simulink model "PVarray_Grid_IncCondReg_det"  (Simulink 10.1)
settings: Solver=FixedStepDiscrete  StartTime=0.0  StopTime=3  RelTol=1e-3
PreLoadFcn:
  | Ts_Power=1e-6
  | Ts_Control=100e-6
undefined symbols (not defined in the file or in its folder): D1, Delta, DiscIntNeverNeededParam, level, sigbuilder_block
libraries: powerlib x29, powerlib_extras x7, simulink x4
(part 2 of 2)

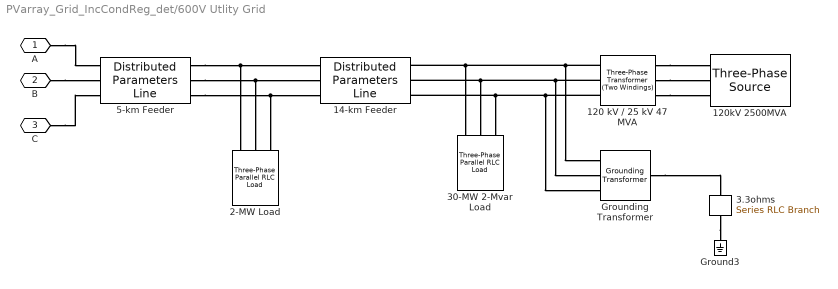
== system PVarray_Grid_IncCondReg_det/600V Utlity Grid ==
  120 kV / 25 kV 47 MVA : powerlib/Elements/Three-Phase Transformer (Two Windings)  Winding1Connection=Yg  Winding2Connection=Delta (D1)  CoreType=Three single-phase transformers  SetSaturation=off  Hysteresis=off  DataFile='basic_model'  SetInitialFlux=off  Measurements=None  UNITS=pu  NominalPower=[47e6 60 ]  Winding1="[ 120e3  0.08/30   0.08 ]"  Winding2="[ 25e3  0.08/30  0.08]"  Rm=500  Lm=500  L0=0.5  Saturation="[ 0,0  ;  0.005,1.2  ;  1.0,1.4 ]"  InitialFluxes=[ 0.8 , -0.8 , 0.7 ]  BreakLoop=off  DiscreteSolver=Trapezoidal iterative  DataType=off  TransfoNumber=0
  120kV 2500MVA : powerlib/Electrical Sources/Three-Phase Source  InternalConnection=Yg  VoltagePhases=off  Voltage=120e3  PhaseAngle=0  Voltage_phases=[25e3 25e3 25e3]/sqrt(3)  PhaseAngles_phases=[0 -120 +120]  Frequency=60  NonIdealSource=on  SpecifyImpedance=on  Resistance=0.8929  Inductance=16.58e-3  ShortCircuitLevel=2500e6  BaseVoltage=120e3  XRratio=7  BusType=swing  Pref=0  Qref=0  Prefabc=[10e3, 10e3, 10e3]  Qrefabc=[0, 0, 0]  Qmin=-inf  Qmax=inf
  14-km Feeder : powerlib/Elements/Distributed Parameters Line  Phases=3  Frequency=60  Resistance=[0.1153 0.413]  Inductance=[1.05e-3 3.32e-3]  Capacitance=[11.33e-009 5.01e-009]  Length=14  x1=[-5.8e-05 -8.79995943472587e-10 0 0;-5.7e-05 -8.80194503979229e-10 0 0;-5.6e-05 -8.80392939390602e-10 0 0;-5.5e-05 -8.80591249678504e-10 0 0;-5.4e-05 -8.80789434814751e-10 0 0;-5.3e-05 -8.80987494771175e-10 0 0;-5.2e-05 -8.8118542951963e-10 0 0;-5.1e-05 -8.81383239031983e-10 0 0;-5e-05 -8.81580923280121e-10 0 0;-4.9e-05 -8.8177848223595e-10 -3790.5008820983 -24060.9143986483;-4.8e-05 -8.81975915871391e-10 -3781.42986192619 -24062.3416739851;-4.7e-05 -8.82173224158384e-10 -3772.35830432856 -24063.7655295266;-4.6e-05 -8.82370407068889e-10 -3763.28621059469 -24065.1859650703;-4.5e-05 -8.8256746457488e-10 -3754.21358201392 -24066.6029804144;-4.4e-05 -8.82764396648352e-10 -3745.14041987568 -24068.0165753574;-4.3e-05 -8.82961203261316e-10 -3736.06672546945 -24069.4267496986;-4.2e-05 -8.83157884385802e-10 -3726.99250008483 -24070.8335032374;-4.1e-05 -8.83354439993856e-10 -3717.91774501146 -24072.236835774;-4e-05 -8.83550870057544e-10 -3708.84246153905 -24073.6367471089;-3.9e-05 -8.83747174548949e-10 -3699.76665095742 -24075.0332370431;-3.8e-05 -8.83943353440171e-10 -3690.69031455644 -24076.4263053782;-3.7e-05 -8.84139406703329e-10 -3681.61345362605 -24077.8159519161;-3.6e-05 -8.8433533431056e-10 -3672.53606945629 -24079.2021764594;-3.5e-05 -8.84531136234017e-10 -3663.45816333725 -24080.5849788111;-3.4e-05 -8.84726812445874e-10 -3654.3797365591 -24081.9643587746;-3.3e-05 -8.84922362918319e-10 -3645.30079041209 -24083.3403161539;-3.2e-05 -8.85117787623562e-10 -3636.22132618654 -24084.7128507535;-3.1e-05 -8.85313086533827e-10 -3627.14134517285 -24086.0819623782;-3e-05 -8.85508259621359e-10 -3618.06084866149 -24087.4476508336;-2.9e-05 -8.85703306858418e-10 -3608.97983794298 -24088.8099159254;-2.8e-05 -8.85898228217286e-10 -3599.89831430796 -24090.1687574601;-2.7e-05 -8.86093023670258e-10 -3590.8162790471 -24091.5241752446;-2.6e-05 -8.86287693189649e-10 -3581.73373345117 -24092.8761690862;-2.5e-05 -8.86482236747794e-10 -3572.65067881099 -24094.2247387928;-2.4e-05 -8.86676654317043e-10 -3563.56711641748 -24095.5698841727;-2.3e-05 -8.86870945869765e-10 -3554.4830475616 -24096.9116050348;-2.2e-05 -8.87065111378347e-10 -3545.39847353442 -24098.2499011883;-2.1e-05 -8.87259150815193e-10 -3536.31339562704 -24099.5847724431;-2e-05 -8.87453064152727e-10 -3527.22781513066 -24100.9162186094;-1.9e-05 -8.87646851363389e-10 -3518.14173333655 -24102.2442394981;-1.8e-05 -8.87840512419637e-10 -3509.05515153604 -24103.5688349203;-1.7e-05 -8.88034047293948e-10 -3499.96807102053 -24104.8900046878;-1.6e-05 -8.88227455958816e-10 -3490.8804930815 -24106.2077486129;-1.5e-05 -8.88420738386753e-10 -3481.79241901051 -24107.5220665083;-1.4e-05 -8.88613894550291e-10 -3472.70385009916 -24108.8329581871;-1.3e-05 -8.88806924421976e-10 -3463.61478763914 -24110.1404234631;-1.2e-05 -8.88999827974376e-10 -3454.52523292222 -24111.4444621504;-1.1e-05 -8.89192605180074e-10 -3445.43518724023 -24112.7450740638;-1e-05 -8.89385256011672e-10 -3436.34465188505 -24114.0422590183;-9e-06 -8.8957778044179e-10 -3427.25362814866 -24115.3360168297;-8e-06 -8.89770178443067e-10 -3418.1621173231 -24116.626347314;-7e-06 -8.89962449988158e-10 -3409.07012070047 -24117.9132502878;-6e-06 -8.90154595049737e-10 -3399.97763957295 -24119.1967255683;-5e-06 -8.90346613600497e-10 -3390.88467523278 -24120.476772973;-4e-06 -8.90538505613146e-10 -3381.79122897228 -24121.7533923201;-3e-06 -8.90730271060413e-10 -3372.69730208382 -24123.026583428;-2e-06 -8.90921909915044e-10 -3363.60289585986 -24124.2963461159;-1e-06 -8.91113422149802e-10 -3354.50801159291 -24125.5626802033]  x2=[-5.8e-05 -9.28142439469267e-10 0 0;-5.7e-05 -9.28357855256912e-10 0 0;-5.6e-05 -9.28573139104203e-10 0 0;-5.5e-05 -9.28788290980541e-10 0 0;-5.4e-05 -9.2900331085535e-10 0 0;-5.3e-05 -9.2921819869807e-10 0 0;-5.2e-05 -9.2943295447816e-10 0 0;-5.1e-05 -9.296475781651e-10 0 0;-5e-05 -9.29862069728387e-10 0 0;-4.9e-05 -9.30076429137536e-10 -3379.33798533185 -24243.9018981732;-4.8e-05 -9.30290656362082e-10 -3370.19800971698 -24245.1741557501;-4.7e-05 -9.30504751371578e-10 -3361.05755512181 -24246.442967547;-4.6e-05 -9.30718714135598e-10 -3351.9166228454 -24247.7083333837;-4.5e-05 -9.30932544623732e-10 -3342.77521418689 -24248.9702530802;-4.4e-05 -9.3114624280559e-10 -3333.63333044547 -24250.2287264573;-4.3e-05 -9.313598086508e-10 -3324.49097292041 -24251.483753336;-4.2e-05 -9.31573242129011e-10 -3315.34814291104 -24252.7353335381;-4.1e-05 -9.31786543209888e-10 -3306.20484171676 -24253.9834668856;-4e-05 -9.31999711863118e-10 -3297.06107063704 -24255.2281532011;-3.9e-05 -9.32212748058403e-10 -3287.91683097141 -24256.4693923078;-3.8e-05 -9.32425651765466e-10 -3278.77212401947 -24257.7071840292;-3.7e-05 -9.3263842295405e-10 -3269.62695108089 -24258.9415281894;-3.6e-05 -9.32851061593915e-10 -3260.4813134554 -24260.1724246131;-3.5e-05 -9.33063567654839e-10 -3251.33521244281 -24261.3998731252;-3.4e-05 -9.33275941106622e-10 -3242.18864934297 -24262.6238735513;-3.3e-05 -9.3348818191908e-10 -3233.04162545582 -24263.8444257174;-3.2e-05 -9.33700290062049e-10 -3223.89414208135 -24265.0615294501;-3.1e-05 -9.33912265505383e-10 -3214.74620051962 -24266.2751845765;-3e-05 -9.34124108218957e-10 -3205.59780207077 -24267.4853909239;-2.9e-05 -9.34335818172662e-10 -3196.44894803497 -24268.6921483205;-2.8e-05 -9.34547395336411e-10 -3187.2996397125 -24269.8954565947;-2.7e-05 -9.34758839680132e-10 -3178.14987840366 -24271.0953155755;-2.6e-05 -9.34970151173776e-10 -3168.99966540885 -24272.2917250923;-2.5e-05 -9.3518132978731e-10 -3159.84900202851 -24273.4846849752;-2.4e-05 -9.3539237549072e-10 -3150.69788956316 -24274.6741950546;-2.3e-05 -9.35603288254013e-10 -3141.54632931337 -24275.8602551614;-2.2e-05 -9.35814068047214e-10 -3132.39432257979 -24277.042865127;-2.1e-05 -9.36024714840365e-10 -3123.24187066312 -24278.2220247835;-2e-05 -9.36235228603529e-10 -3114.08897486412 -24279.3977339632;-1.9e-05 -9.36445609306788e-10 -3104.93563648363 -24280.5699924989;-1.8e-05 -9.36655856920241e-10 -3095.78185682254 -24281.7388002242;-1.7e-05 -9.36865971414008e-10 -3086.62763718181 -24282.9041569729;-1.6e-05 -9.37075952758227e-10 -3077.47297886245 -24284.0660625793;-1.5e-05 -9.37285800923054e-10 -3068.31788316555 -24285.2245168784;-1.4e-05 -9.37495515878667e-10 -3059.16235139226 -24286.3795197055;-1.3e-05 -9.37705097595258e-10 -3050.00638484376 -24287.5310708964;-1.2e-05 -9.37914546043043e-10 -3040.84998482134 -24288.6791702875;-1.1e-05 -9.38123861192253e-10 -3031.69315262632 -24289.8238177156;-1e-05 -9.38333043013142e-10 -3022.53588956009 -24290.965013018;-9e-06 -9.38542091475978e-10 -3013.3781969241 -24292.1027560326;-8e-06 -9.38751006551052e-10 -3004.22007601987 -24293.2370465976;-7e-06 -9.38959788208673e-10 -2995.06152814897 -24294.3678845519;-6e-06 -9.39168436419167e-10 -2985.90255461302 -24295.4952697347;-5e-06 -9.39376951152881e-10 -2976.74315671374 -24296.6192019857;-4e-06 -9.39585332380181e-10 -2967.58333575286 -24297.7396811453;-3e-06 -9.39793580071451e-10 -2958.42309303221 -24298.8567070543;-2e-06 -9.40001694197093e-10 -2949.26242985367 -24299.9702795538;-1e-06 -9.40209674727532e-10 -2940.10134751915 -24301.0803984855]  x3=[-5.8e-05 5.3332967211062e-13 0 0;-5.7e-05 5.31949059499138e-13 0 0;-5.6e-05 5.30568371285831e-13 0 0;-5.5e-05 5.29187607666925e-13 0 0;-5.4e-05 5.27806768838659e-13 0 0;-5.3e-05 5.2642585499728e-13 0 0;-5.2e-05 5.25044866339047e-13 0 0;-5.1e-05 5.23663803060229e-13 0 0;-5e-05 5.22282665357106e-13 0 0;-4.9e-05 5.20901453425968e-13 -23.6102100346326 -155.666879550863;-4.8e-05 5.19520167463117e-13 -23.5515233272294 -155.675769328272;-4.7e-05 5.18138807664864e-13 -23.4928332726296 -155.684636980683;-4.6e-05 5.16757374227531e-13 -23.4341398791742 -155.693482506834;-4.5e-05 5.15375867347451e-13 -23.3754431552049 -155.702305905469;-4.4e-05 5.13994287220966e-13 -23.3167431090639 -155.711107175334;-4.3e-05 5.1261263404443e-13 -23.2580397490936 -155.719886315178;-4.2e-05 5.11230908014206e-13 -23.1993330836372 -155.728643323754;-4.1e-05 5.09849109326669e-13 -23.1406231210382 -155.737378199816;-4e-05 5.08467238178203e-13 -23.0819098696406 -155.746090942124;-3.9e-05 5.07085294765203e-13 -23.0231933377888 -155.754781549438;-3.8e-05 5.05703279284074e-13 -22.9644735338277 -155.763450020525;-3.7e-05 5.04321191931231e-13 -22.9057504661029 -155.772096354151;-3.6e-05 5.02939032903099e-13 -22.84702414296 -155.780720549089;-3.5e-05 5.01556802396114e-13 -22.7882945727455 -155.789322604112;-3.4e-05 5.00174500606722e-13 -22.7295617638061 -155.797902517998;-3.3e-05 4.98792127731378e-13 -22.6708257244891 -155.806460289528;-3.2e-05 4.9740968396655e-13 -22.6120864631422 -155.814995917485;-3.1e-05 4.96027169508712e-13 -22.5533439881135 -155.823509400656;-3e-05 4.94644584554351e-13 -22.4945983077516 -155.832000737831;-2.9e-05 4.93261929299964e-13 -22.4358494304056 -155.840469927803;-2.8e-05 4.91879203942055e-13 -22.3770973644251 -155.848916969369;-2.7e-05 4.90496408677142e-13 -22.31834211816 -155.857341861329;-2.6e-05 4.8911354370175e-13 -22.2595836999608 -155.865744602484;-2.5e-05 4.87730609212416e-13 -22.2008221181782 -155.874125191641;-2.4e-05 4.86347605405685e-13 -22.1420573811638 -155.882483627608;-2.3e-05 4.84964532478113e-13 -22.0832894972691 -155.890819909198;-2.2e-05 4.83581390626265e-13 -22.0245184748466 -155.899134035226;-2.1e-05 4.82198180046717e-13 -21.9657443222488 -155.90742600451;-2e-05 4.80814900936054e-13 -21.9069670478288 -155.915695815872;-1.9e-05 4.79431553490871e-13 -21.8481866599403 -155.923943468137;-1.8e-05 4.78048137907771e-13 -21.7894031669371 -155.932168960131;-1.7e-05 4.7666465438337e-13 -21.7306165771739 -155.940372290687;-1.6e-05 4.75281103114291e-13 -21.6718268990054 -155.948553458638;-1.5e-05 4.73897484297168e-13 -21.613034140787 -155.956712462822;-1.4e-05 4.72513798128643e-13 -21.5542383108744 -155.964849302079;-1.3e-05 4.7113004480537e-13 -21.4954394176239 -155.972963975253;-1.2e-05 4.6974622452401e-13 -21.436637469392 -155.98105648119;-1.1e-05 4.68362337481236e-13 -21.3778324745359 -155.98912681874;-1e-05 4.66978383873729e-13 -21.319024441413 -155.997174986756;-9e-06 4.65594363898178e-13 -21.2602133783814 -156.005200984095;-8e-06 4.64210277751285e-13 -21.2013992937992 -156.013204809616;-7e-06 4.62826125629759e-13 -21.1425821960254 -156.021186462181;-6e-06 4.61441907730319e-13 -21.0837620934191 -156.029145940655;-5e-06 4.60057624249692e-13 -21.02493899434 -156.037083243909;-4e-06 4.58673275384617e-13 -20.9661129071483 -156.044998370812;-3e-06 4.57288861331841e-13 -20.9072838402043 -156.052891320242;-2e-06 4.55904382288119e-13 -20.8484518018689 -156.060762091076;-1e-06 4.54519838450217e-13 -20.7896168005037 -156.068610682194]  x4=[-5.8e-05 -2.65449914026147e-12 0 0;-5.7e-05 -2.65328779442914e-12 0 0;-5.6e-05 -2.65207607150545e-12 0 0;-5.5e-05 -2.65086397166259e-12 0 0;-5.4e-05 -2.64965149507285e-12 0 0;-5.3e-05 -2.64843864190854e-12 0 0;-5.2e-05 -2.64722541234203e-12 0 0;-5.1e-05 -2.64601180654575e-12 0 0;-5e-05 -2.64479782469219e-12 0 0;-4.9e-05 -2.64358346695387e-12 -1.28892375628919 -2.16547060902834;-4.8e-05 -2.64236873350338e-12 -1.28810730152929 -2.16595636794445;-4.7e-05 -2.64115362451337e-12 -1.28729066370062 -2.16644181902986;-4.6e-05 -2.63993814015653e-12 -1.28647384291924 -2.16692696221557;-4.5e-05 -2.6387222806056e-12 -1.28565683930124 -2.16741179743263;-4.4e-05 -2.63750604603338e-12 -1.28483965296273 -2.16789632461214;-4.3e-05 -2.63628943661274e-12 -1.28402228401984 -2.16838054368524;-4.2e-05 -2.63507245251657e-12 -1.28320473258876 -2.1688644545831;-4.1e-05 -2.63385509391785e-12 -1.28238699878567 -2.16934805723695;-4e-05 -2.63263736098957e-12 -1.28156908272678 -2.16983135157806;-3.9e-05 -2.63141925390481e-12 -1.28075098452835 -2.17031433753775;-3.8e-05 -2.63020077283669e-12 -1.27993270430663 -2.17079701504737;-3.7e-05 -2.62898191795839e-12 -1.27911424217794 -2.17127938403832;-3.6e-05 -2.62776268944312e-12 -1.27829559825858 -2.17176144444204;-3.5e-05 -2.62654308746417e-12 -1.27747677266492 -2.17224319619003;-3.4e-05 -2.62532311219487e-12 -1.27665776551331 -2.17272463921382;-3.3e-05 -2.62410276380861e-12 -1.27583857692017 -2.17320577344498;-3.2e-05 -2.62288204247882e-12 -1.2750192070019 -2.17368659881513;-3.1e-05 -2.621660948379e-12 -1.27419965587498 -2.17416711525595;-3e-05 -2.6204394816827e-12 -1.27337992365586 -2.17464732269912;-2.9e-05 -2.6192176425635e-12 -1.27256001046106 -2.17512722107642;-2.8e-05 -2.61799543119506e-12 -1.27173991640711 -2.17560681031962;-2.7e-05 -2.61677284775108e-12 -1.27091964161055 -2.17608609036058;-2.6e-05 -2.61554989240533e-12 -1.27009918618796 -2.17656506113118;-2.5e-05 -2.6143265653316e-12 -1.26927855025595 -2.17704372256334;-2.4e-05 -2.61310286670377e-12 -1.26845773393116 -2.17752207458904;-2.3e-05 -2.61187879669574e-12 -1.26763673733023 -2.17800011714028;-2.2e-05 -2.61065435548148e-12 -1.26681556056985 -2.17847785014914;-2.1e-05 -2.60942954323502e-12 -1.26599420376673 -2.17895527354771;-2e-05 -2.60820436013043e-12 -1.2651726670376 -2.17943238726814;-1.9e-05 -2.60697880634183e-12 -1.26435095049922 -2.17990919124262;-1.8e-05 -2.6057528820434e-12 -1.26352905426837 -2.18038568540339;-1.7e-05 -2.60452658740937e-12 -1.26270697846186 -2.18086186968273;-1.6e-05 -2.60329992261403e-12 -1.26188472319653 -2.18133774401296;-1.5e-05 -2.60207288783172e-12 -1.26106228858924 -2.18181330832645;-1.4e-05 -2.60084548323681e-12 -1.26023967475687 -2.18228856255561;-1.3e-05 -2.59961770900376e-12 -1.25941688181634 -2.1827635066329;-1.2e-05 -2.59838956530706e-12 -1.25859390988459 -2.18323814049082;-1.1e-05 -2.59716105232125e-12 -1.25777075907857 -2.1837124640619;-1e-05 -2.59593217022093e-12 -1.25694742951527 -2.18418647727874;-9e-06 -2.59470291918076e-12 -1.25612392131172 -2.18466018007397;-8e-06 -2.59347329937544e-12 -1.25530023458494 -2.18513357238027;-7e-06 -2.59224331097972e-12 -1.254476369452 -2.18560665413036;-6e-06 -2.59101295416842e-12 -1.25365232602999 -2.186079425257;-5e-06 -2.58978222911639e-12 -1.25282810443603 -2.186551885693;-4e-06 -2.58855113599855e-12 -1.25200370478726 -2.18702403537121;-3e-06 -2.58731967498987e-12 -1.25117912720083 -2.18749587422453;-2e-06 -2.58608784626536e-12 -1.25035437179395 -2.18796740218591;-1e-06 -2.58485565000009e-12 -1.24952943868383 -2.18843861918832]  x5=5.70973484498186e-05  V1=ones(3,3)  V2=ones(3,3)  I1=ones(3,3)  I2=ones(3,3)  nHarmo=1  Measurements=None
  2-MW Load : powerlib/Elements/Three-Phase Parallel RLC Load  LConnTagsString=A|B|C  Configuration=Y (grounded)  NominalVoltage=25e3  Vabc=[1e3 1e3 1e3]  Vabcp=[1e3 1e3 1e3]  NominalFrequency=60  UnbalancedPower=off  ActivePower=2e6  InductivePower=0  CapacitivePower=0  Pabc=[10e3 9e3 11e3]  QLabc=[100 90 110]  QCabc=[100 90 110]  Pabcp=[10e3 9e3 11e3]  QLabcp=[100 90 110]  QCabcp=[100 90 110]  Measurements=None  LoadType=constant Z
  "3.3ohms " : powerlib/Elements/Series RLC Branch  LConnTagsString=__new0  RConnTagsString=__new0  BranchType=R  Resistance=3.3  Inductance=[]  SetiL0=off  InitialCurrent=0  Capacitance=[]  Setx0=off  InitialVoltage=0  Measurements=None
  30-MW 2-Mvar Load : powerlib/Elements/Three-Phase Parallel RLC Load  LConnTagsString=A|B|C  Configuration=Y (grounded)  NominalVoltage=25e3  Vabc=[1e3 1e3 1e3]  Vabcp=[1e3 1e3 1e3]  NominalFrequency=60  UnbalancedPower=off  ActivePower=30e6  InductivePower=2e6  CapacitivePower=0  Pabc=[10e3 9e3 11e3]  QLabc=[100 90 110]  QCabc=[100 90 110]  Pabcp=[10e3 9e3 11e3]  QLabcp=[100 90 110]  QCabcp=[100 90 110]  Measurements=None  LoadType=constant Z
  5-km Feeder : powerlib/Elements/Distributed Parameters Line  Phases=3  Frequency=60  Resistance=[0.1153 0.413]  Inductance=[1.05e-3 3.32e-3]  Capacitance=[11.33e-009 5.01e-009]  Length=5  x1=[-2.1e-05 -8.79160357709828e-10 -3536.88834564081 -24100.782456774;-2e-05 -8.79350132865022e-10 -3527.80231358723 -24102.1141196063;-1.9e-05 -8.79539783044952e-10 -3518.71578015427 -24103.4423569906;-1.8e-05 -8.79729308222663e-10 -3509.62874663332 -24104.7671687382;-1.7e-05 -8.79918708371221e-10 -3500.54121431586 -24106.0885546609;-1.6e-05 -8.80107983463706e-10 -3491.45318449342 -24107.4065145707;-1.5e-05 -8.80297133473218e-10 -3482.36465845762 -24108.7210482804;-1.4e-05 -8.80486158372876e-10 -3473.27563750013 -24110.0321556032;-1.3e-05 -8.80675058135815e-10 -3464.18612291272 -24111.3398363528;-1.2e-05 -8.80863832735187e-10 -3455.09611598721 -24112.6440903432;-1.1e-05 -8.81052482144163e-10 -3446.00561801548 -24113.9449173892;-1e-05 -8.81241006335934e-10 -3436.9146302895 -24115.2423173058;-9e-06 -8.81429405283703e-10 -3427.82315410131 -24116.5362899086;-8e-06 -8.81617678960698e-10 -3418.73119074299 -24117.8268350139;-7e-06 -8.81805827340158e-10 -3409.63874150674 -24119.113952438;-6e-06 -8.81993850395344e-10 -3400.54580768477 -24120.3976419982;-5e-06 -8.82181748099535e-10 -3391.45239056941 -24121.6779035119;-4e-06 -8.82369520426025e-10 -3382.35849145303 -24122.9547367972;-3e-06 -8.82557167348127e-10 -3373.26411162807 -24124.2281416727;-2e-06 -8.82744688839174e-10 -3364.16925238706 -24125.4981179574;-1e-06 -8.82932084872514e-10 -3355.07391502257 -24126.7646654707]  x2=[-2.1e-05 -8.87264550983724e-10 -3536.31339562704 -24099.5847724431;-2e-05 -8.8745820717537e-10 -3527.22781513066 -24100.9162186094;-1.9e-05 -8.87651737239413e-10 -3518.14173333655 -24102.2442394981;-1.8e-05 -8.87845141148348e-10 -3509.05515153604 -24103.5688349203;-1.7e-05 -8.88038418874688e-10 -3499.96807102053 -24104.8900046878;-1.6e-05 -8.88231570390964e-10 -3490.8804930815 -24106.2077486129;-1.5e-05 -8.88424595669725e-10 -3481.79241901051 -24107.5220665083;-1.4e-05 -8.88617494683537e-10 -3472.70385009916 -24108.8329581871;-1.3e-05 -8.88810267404986e-10 -3463.61478763914 -24110.1404234631;-1.2e-05 -8.89002913806674e-10 -3454.52523292222 -24111.4444621504;-1.1e-05 -8.89195433861221e-10 -3445.43518724023 -24112.7450740638;-1e-05 -8.89387827541267e-10 -3436.34465188505 -24114.0422590183;-9e-06 -8.89580094819467e-10 -3427.25362814866 -24115.3360168297;-8e-06 -8.89772235668497e-10 -3418.1621173231 -24116.626347314;-7e-06 -8.89964250061049e-10 -3409.07012070047 -24117.9132502878;-6e-06 -8.90156137969833e-10 -3399.97763957295 -24119.1967255683;-5e-06 -8.90347899367578e-10 -3390.88467523278 -24120.476772973;-4e-06 -8.9053953422703e-10 -3381.79122897228 -24121.7533923201;-3e-06 -8.90731042520954e-10 -3372.69730208382 -24123.026583428;-2e-06 -8.90922424222132e-10 -3363.60289585986 -24124.2963461159;-1e-06 -8.91113679303365e-10 -3354.50801159291 -24125.5626802033]  x3=[-2.1e-05 7.49995944592519e-13 -11.223690275522 -79.1234381044518;-2e-05 7.48413306611119e-13 -11.1938606452351 -79.1276637132989;-1.9e-05 7.46830562263496e-13 -11.164029424051 -79.1318780763402;-1.8e-05 7.45247711774596e-13 -11.1341966162093 -79.136081192977;-1.7e-05 7.43664755369375e-13 -11.10436222595 -79.1402730626117;-1.6e-05 7.42081693272807e-13 -11.0745262575131 -79.1444536846487;-1.5e-05 7.40498525709882e-13 -11.0446887151391 -79.1486230584937;-1.4e-05 7.38915252905601e-13 -11.0148496030685 -79.1527811835543;-1.3e-05 7.37331875084984e-13 -10.9850089255421 -79.1569280592394;-1.2e-05 7.35748392473064e-13 -10.955166686801 -79.1610636849597;-1.1e-05 7.34164805294888e-13 -10.9253228910864 -79.1651880601274;-1e-05 7.32581113775521e-13 -10.8954775426397 -79.1693011841564;-9e-06 7.3099731814004e-13 -10.8656306457027 -79.1734030564621;-8e-06 7.29413418613537e-13 -10.8357822045173 -79.1774936764615;-7e-06 7.2782941542112e-13 -10.8059322233255 -79.1815730435733;-6e-06 7.26245308787912e-13 -10.7760807063698 -79.1856411572176;-5e-06 7.24661098939049e-13 -10.7462276578927 -79.1896980168164;-4e-06 7.23076786099682e-13 -10.716373082137 -79.193743621793;-3e-06 7.21492370494978e-13 -10.6865169833457 -79.1977779715724;-2e-06 7.19907852350118e-13 -10.6566593657619 -79.2018010655814;-1e-06 7.18323231890297e-13 -10.6268002336293 -79.2058129032482]  x4=[-2.1e-05 -2.89139379379673e-12 -12.4922083172321 -78.9091123636669;-2e-05 -2.89090994973168e-12 -12.4624593957017 -78.9138162077682;-1.9e-05 -2.89042569480385e-12 -12.4327087029779 -78.9185088364563;-1.8e-05 -2.88994102908207e-12 -12.4029562432888 -78.9231902490643;-1.7e-05 -2.88945595263521e-12 -12.3732020208632 -78.9278604449268;-1.6e-05 -2.88897046553223e-12 -12.3434460399295 -78.9325194233801;-1.5e-05 -2.88848456784211e-12 -12.3136883047169 -78.9371671837621;-1.4e-05 -2.88799825963392e-12 -12.2839288194546 -78.9418037254122;-1.3e-05 -2.88751154097677e-12 -12.254167588372 -78.9464290476714;-1.2e-05 -2.88702441193984e-12 -12.2244046156989 -78.9510431498825;-1.1e-05 -2.88653687259235e-12 -12.1946399056653 -78.9556460313895;-1e-05 -2.88604892300359e-12 -12.1648734625014 -78.9602376915384;-9e-06 -2.88556056324292e-12 -12.1351052904377 -78.9648181296766;-8e-06 -2.88507179337974e-12 -12.1053353937049 -78.9693873451531;-7e-06 -2.88458261348351e-12 -12.075563776534 -78.9739453373185;-6e-06 -2.88409302362377e-12 -12.0457904431561 -78.978492105525;-5e-06 -2.88360302387009e-12 -12.0160153978028 -78.9830276491264;-4e-06 -2.8831126142921e-12 -11.9862386447058 -78.9875519674782;-3e-06 -2.88262179495952e-12 -11.9564601880969 -78.9920650599372;-2e-06 -2.88213056594209e-12 -11.9266800322083 -78.9965669258622;-1e-06 -2.88163892730964e-12 -11.8968981812726 -79.0010575646132]  x5=2.03919101606495e-05  V1=ones(3,3)  V2=ones(3,3)  I1=ones(3,3)  I2=ones(3,3)  nHarmo=1  Measurements=None
  Ground3 : powerlib/Elements/Ground  LConnTagsString=a
  "Grounding Transformer " : powerlib/Elements/Grounding Transformer   UNITS=pu  NominalPower="[100e6   60]"  NominalVoltage=25e3  ZeroSequenceImpedance_pu=[0.025 0.75]  MagnetizationBranch_pu=[500 500]  ZeroSequenceImpedance_SI=[0.052083 589.05]  MagnetizationBranch_SI=[1041.7 3.927e+005]  Measurements=None
      settings: SourceProductBaseCode=PS
  A : PMIOPort  Side=Left
  B : PMIOPort  Port=2  Side=Left
  C : PMIOPort  Port=3  Side=Left
  connections:
  "3.3ohms "/RConn1 -- Ground3/LConn1
  120 kV / 25 kV 47 MVA/LConn1 -- 120kV 2500MVA/RConn1
  120 kV / 25 kV 47 MVA/LConn2 -- 120kV 2500MVA/RConn2
  120 kV / 25 kV 47 MVA/LConn3 -- 120kV 2500MVA/RConn3
  120 kV / 25 kV 47 MVA/RConn1 -- "Grounding Transformer "/LConn1 -- 14-km Feeder/RConn1 -- 30-MW 2-Mvar Load/LConn1
  120 kV / 25 kV 47 MVA/RConn2 -- "Grounding Transformer "/LConn2 -- 14-km Feeder/RConn2 -- 30-MW 2-Mvar Load/LConn2
  120 kV / 25 kV 47 MVA/RConn3 -- "Grounding Transformer "/LConn3 -- 14-km Feeder/RConn3 -- 30-MW 2-Mvar Load/LConn3
  5-km Feeder/RConn1 -- 14-km Feeder/LConn1 -- 2-MW Load/LConn1
  5-km Feeder/RConn2 -- 14-km Feeder/LConn2 -- 2-MW Load/LConn2
  5-km Feeder/RConn3 -- 14-km Feeder/LConn3 -- 2-MW Load/LConn3
  A/RConn1 -- 5-km Feeder/LConn1
  B/RConn1 -- 5-km Feeder/LConn2
  C/RConn1 -- 5-km Feeder/LConn3
  "Grounding Transformer "/RConn1 -- "3.3ohms "/LConn1

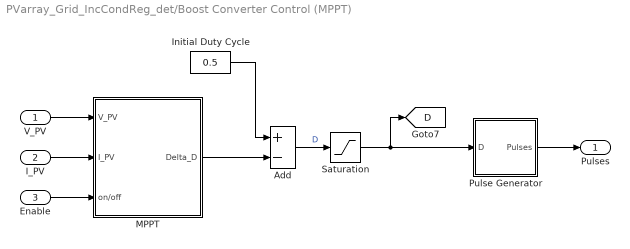
== system PVarray_Grid_IncCondReg_det/Boost Converter Control (MPPT) ==
  V_PV : Inport
  I_PV : Inport  Port=2
  Enable : Inport  Port=3
  Add : Sum  Inputs=+-
  Initial Duty Cycle : Constant  Value=0.5
  MPPT : Subsystem
  Pulse Generator : Subsystem  mask{Freq=5000}
      mask prompts: Freq "Frequency (Hz)"
  Saturation : Saturate  UpperLimit=1  LowerLimit=0
  Pulses : Outport
  tag scope: D=global
  wires:
  Initial Duty Cycle/1 -> Add/1
  MPPT/1(Delta_D) -> Add/2
  Add/1 -> Saturation/1  "D"
  Saturation/1 -> Pulse Generator/1(D), [D]
  Enable/1 -> MPPT/3(on/off)
  Pulse Generator/1(Pulses) -> Pulses/1
  I_PV/1 -> MPPT/2(I_PV)
  V_PV/1 -> MPPT/1(V_PV)

== system PVarray_Grid_IncCondReg_det/Irradiance (W/m2)  ==
  Demux : Demux  Tag=STV Demux  Outputs=1
      settings: DisplayOption=none
  FromWs : FromWorkspace  Tag=STV FromWs  VariableName=tuvar  SigBuilderData=DataTag0  VnvData=DataTag1
      SigBuilderData=|
      | common.afterFinalStr = 'Extrapolate'
      | common.sampleTime = '0'
      | dataSet(1).timeRange = [0 1]
      | dataSet(1).name = 'Constant Irradiance'
      | dataSet(2).timeRange = [0 1]
      | dataSet(2).name = 'Step Irradiance'
      | dataSet(3).timeRange = [0 3]
      | dataSet(3).name = 'Ramp-up/down Irradiance'
      | sbobj.Groups(1).Name = 'Constant Irradiance'
      | sbobj.Groups(1).Signals.Name = 'Ir'
      | sbobj.Groups(1).Signals.XData = [0 1]
      | sbobj.Groups(1).Signals.YData = [1000 1000]
      | sbobj.Groups(1).TimeRange = [0 1]
      | sbobj.Groups(2).Name = 'Step Irradiance'
      | sbobj.Groups(2).Signals.Name = 'Ir'
      | sbobj.Groups(2).Signals.XData = [0 0.501 0.51 0.69 0.7 1]
      | sbobj.Groups(2).Signals.YData = [1000 1000 250 250 1000 1000]
      | sbobj.Groups(2).TimeRange = [0 1]
      | sbobj.Groups(3).Name = 'Ramp-up/down Irradiance'
      | sbobj.Groups(3).Signals.Name = 'Ir'
      | sbobj.Groups(3).Signals.XData = [0 0.7 1.2 1.5 2 2.3 2.35 2.65 2.7 3]
      | sbobj.Groups(3).Signals.YData = [1000 1000 250 250 1000 1000 250 250 1000 1000]
      | sbobj.Groups(3).TimeRange = [0 3]
  Ir : Outport  Tag=STV Outport
  wires:
  Demux/1 -> Ir/1
  FromWs/1 -> Demux/1

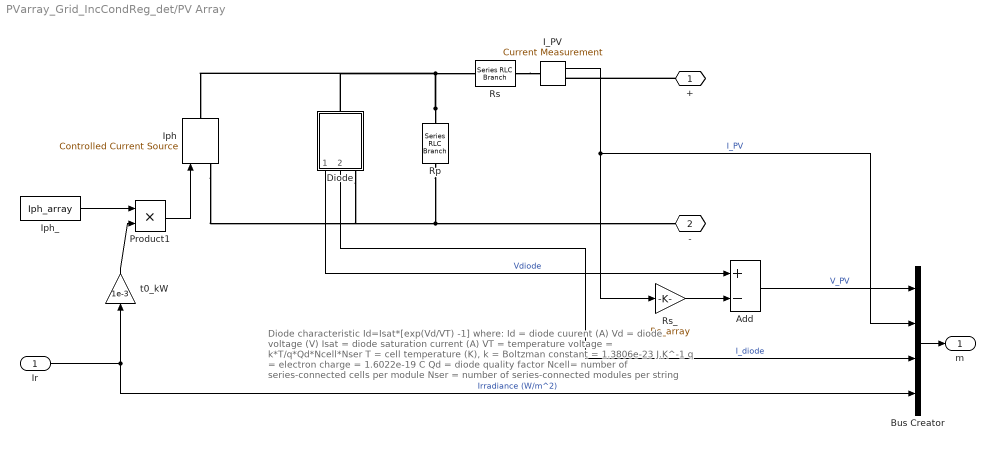
== system PVarray_Grid_IncCondReg_det/PV Array ==
  note: Diode characteristic
      |    Id=Isat*[exp(Vd/VT) -1]
      |
      | where:
      |    Id = diode cuurent (A)
      |    Vd = diode voltage (V)
      |  Isat = diode saturation current (A)
      |    VT = temperature voltage = k*T/q*Qd*Ncell*Nser
      |
      |     T = cell temperature (K),
      |     k = Boltzman constant = 1.3806e-23 J.K^-1
      |     q = electron charge = 1.6022e-19 C
      |    Qd = diode quality factor
      |  Ncell= number of series-connected cells per module
      |  Nser = number of series-connected modules per string
  Ir : Inport
  Add : Sum  Inputs=+-
  Bus Creator : BusCreator  Inputs=4
  Diode : Subsystem
      mask Display:
      | plot(-75,-50,100,150, [-15 -15 43 -15 -15 -75],[50 8 50 92 50 50], ...
      |     [43 43],[8 94],[100 43], [50 50])
  I_PV : powerlib/Measurements/Current Measurement  PhasorSimulation=off  OutputType=Complex  PSBequivalent=0
  Iph : powerlib/Electrical Sources/Controlled Current Source  Initialize=on  Source_Type=AC  Amplitude=0  Phase=0  Frequency=0  Measurements=None
  Iph_ : Constant  Value=Iph_array
  Product1 : Product  Inputs=**  RndMeth=Zero
  Rp : powerlib/Elements/Series RLC Branch  LConnTagsString=__new0  RConnTagsString=__new0  BranchType=R  Resistance=Rp_array  Inductance=1e-3  SetiL0=off  InitialCurrent=0  Capacitance=1e-6  Setx0=off  InitialVoltage=0  Measurements=Branch current
  Rs : powerlib/Elements/Series RLC Branch  LConnTagsString=__new0  RConnTagsString=__new0  BranchType=R  Resistance=Rs_array  Inductance=1e-3  SetiL0=off  InitialCurrent=0  Capacitance=1e-6  Setx0=off  InitialVoltage=0  Measurements=None
  Rs_ : Gain  Gain=Rs_array
  t0_kW : Gain  Gain=1e-3
  + : PMIOPort  Side=Right
  - : PMIOPort  Port=2  Side=Right
  m : Outport
  wires:
  Bus Creator/1 -> m/1
  Diode/2(Idiode) -> Bus Creator/3  "I_diode"
  Add/1 -> Bus Creator/1  "V_PV"
  t0_kW/1 -> Product1/2
  I_PV/1 -> Bus Creator/2, Rs_/1  "I_PV"
  Rs_/1 -> Add/2
  Diode/1(Vdiode) -> Add/1  "Vdiode"
  Ir/1 -> Bus Creator/4, t0_kW/1  "Irradiance (W/m^2)"
  Iph_/1 -> Product1/1
  Product1/1 -> Iph/1
  connections:
  +/RConn1 -- I_PV/RConn1
  Rs/LConn1 -- I_PV/LConn1
  Rp/LConn1 -- Rs/RConn1 -- Iph/RConn1 -- Diode/LConn1
  Rp/RConn1 -- -/RConn1 -- Diode/RConn1 -- Iph/LConn1

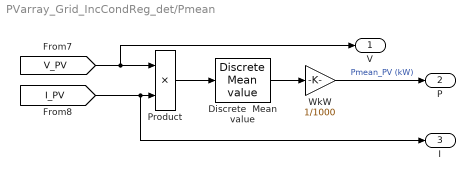
== system PVarray_Grid_IncCondReg_det/Pmean ==
  Discrete  Mean value : powerlib_extras/Discrete Measurements/Discrete  Mean value  Freq=60  Vinit=0  Ts=Ts_Control
      settings: SourceProductBaseCode=PS
  Product : Product  RndMeth=Zero
  WkW : Gain  Gain=1/1000
  V : Outport
  P : Outport  Port=2
  I : Outport  Port=3
  wires:
  [V_PV] -> Product/1, V/1
  Product/1 -> Discrete  Mean value/1
  [I_PV] -> I/1, Product/2
  WkW/1 -> P/1  "Pmean_PV (kW)"
  Discrete  Mean value/1 -> WkW/1

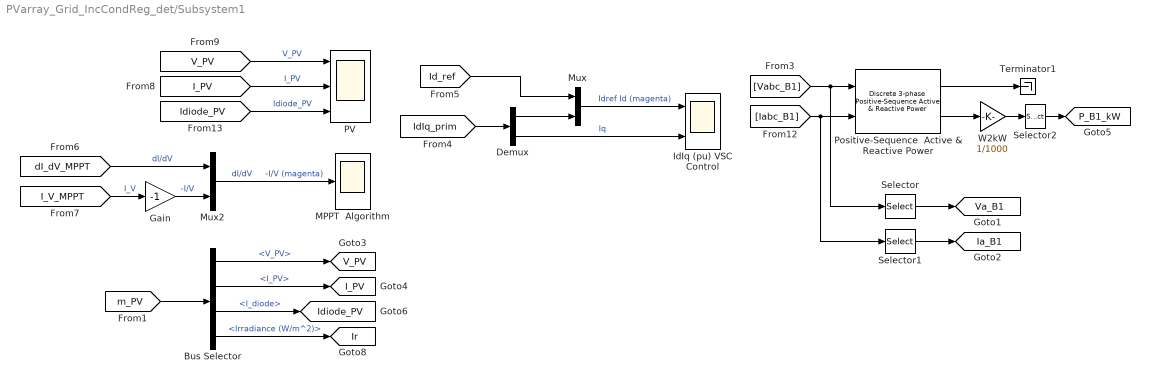
== system PVarray_Grid_IncCondReg_det/Subsystem1 ==
  Bus Selector : BusSelector  OutputSignals=V_PV,I_PV,I_diode,Irradiance (W/m^2)
  Demux : Demux  Outputs=2
  Gain : Gain  Gain=-1
  IdIq (pu) VSC Control : Scope  NumInputPorts=2
  MPPT  Algorithm : Scope
  Mux : Mux  Inputs=2
  Mux2 : Mux  Inputs=2
  PV : Scope  NumInputPorts=3
  Positive-Sequence  Active & Reactive Power : powerlib_extras/Discrete Measurements/Discrete 3-phase  Positive-Sequence  Active & Reactive Power  Freq=60  Par_Vinit=[0 0]  Par_Iinit=[0 0]  Ts=Ts_Control
      settings: SourceProductBaseCode=PS
  Selector : Selector  InputPortWidth=3  IndexOptions=Index vector (dialog)  Indices=[1]  OutputSizes=1
  Selector1 : Selector  InputPortWidth=3  IndexOptions=Index vector (dialog)  Indices=[1]  OutputSizes=1
  Selector2 : Selector  InputPortWidth=2  IndexOptions=Index vector (dialog)  Indices=[1]  OutputSizes=1
  Terminator1 : Terminator
  W2kW : Gain  Gain=1/1000
  tag scope: I_PV=global, Ia_B1=global, Idiode_PV=global, Ir=global, P_B1_kW=global, V_PV=global, Va_B1=global
  wires:
  [Vabc_B1] -> Positive-Sequence  Active & Reactive Power/1, Selector/1
  [Iabc_B1] -> Positive-Sequence  Active & Reactive Power/2, Selector1/1
  Positive-Sequence  Active & Reactive Power/2 -> W2kW/1
  Positive-Sequence  Active & Reactive Power/1 -> Terminator1/1
  W2kW/1 -> Selector2/1
  [I_V_MPPT] -> Gain/1  "I_V"
  [IdIq_prim] -> Demux/1
  [Id_ref] -> Mux/1
  Demux/1 -> Mux/2
  Mux/1 -> IdIq (pu) VSC Control/1  "Idref Id (magenta)"
  Demux/2 -> IdIq (pu) VSC Control/2  "Iq"
  Selector/1 -> [Va_B1]
  Selector1/1 -> [Ia_B1]
  [V_PV] -> PV/1  "V_PV"
  [I_PV] -> PV/2  "I_PV"
  [Idiode_PV] -> PV/3  "Idiode_PV"
  [dI_dV_MPPT] -> Mux2/1  "dI/dV"
  Gain/1 -> Mux2/2  "-I/V"
  Mux2/1 -> MPPT  Algorithm/1  "dI/dV     -I/V (magenta)"
  Selector2/1 -> [P_B1_kW]
  [m_PV] -> Bus Selector/1
  Bus Selector/1 -> [V_PV]  "<V_PV>"
  Bus Selector/2 -> [I_PV]  "<I_PV>"
  Bus Selector/3 -> [Idiode_PV]  "<I_diode>"
  Bus Selector/4 -> [Ir]  "<Irradiance (W/m^2)>"

== system PVarray_Grid_IncCondReg_det/Subsystem2 ==
  Discrete  Mean value : powerlib_extras/Discrete Measurements/Discrete  Mean value  Freq=60  Vinit=0  Ts=Ts_Control
      settings: SourceProductBaseCode=PS
  Mux1 : Mux  Inputs=2
  Vm : Outport
  "Vdc " : Outport  Port=2
  wires:
  [Vdc_ref] -> Mux1/1  "Vdc ref"
  [Vdc] -> Discrete  Mean value/1  "Vdc"
  Mux1/1 -> "Vdc "/1
  Discrete  Mean value/1 -> Mux1/2, Vm/1

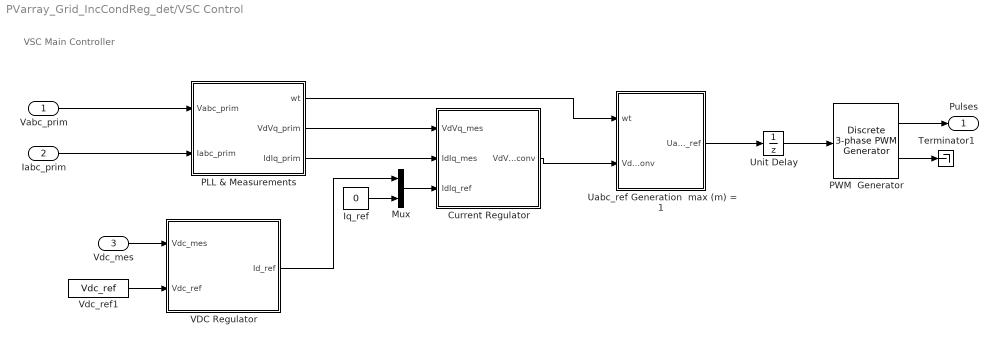
== system PVarray_Grid_IncCondReg_det/VSC Control ==
  note: VSC Main Controller
  Vabc_prim : Inport  PortDimensions=3
  Iabc_prim : Inport  Port=2  PortDimensions=3
  Vdc_mes : Inport  Port=3  PortDimensions=1
  Current Regulator : Subsystem
  Iq_ref : Constant  Value=0
  Mux : Mux  Inputs=2
  PLL & Measurements : Subsystem
  PWM  Generator : powerlib_extras/Discrete  Control Blocks/Discrete 3-phase PWM Generator  ModulatorType=3-level  ModulatorMode=Un-synchronized  nF=18  Fc=33*60  ModulatingSignals=off  m=0.2  Freq=60  Phase=0  Ts=Ts_Power
      settings: SourceProductBaseCode=PS
  Terminator1 : Terminator
  Uabc_ref Generation  max (m) = 1 : Subsystem
  Unit Delay : UnitDelay  SampleTime=Ts_Control  HasFrameUpgradeWarning=on
  VDC Regulator : Subsystem
  Vdc_ref1 : Constant  Value=Vdc_ref
  Pulses : Outport
  wires:
  VDC Regulator/1(Id_ref) -> Mux/1
  PLL & Measurements/1(wt) -> Uabc_ref Generation  max (m) = 1/1(wt)
  Current Regulator/1(VdVq_conv) -> Uabc_ref Generation  max (m) = 1/2(VdVq_conv)
  Iq_ref/1 -> Mux/2
  Mux/1 -> Current Regulator/3(IdIq_ref)
  PLL & Measurements/3(IdIq_prim) -> Current Regulator/2(IdIq_mes)
  PLL & Measurements/2(VdVq_prim) -> Current Regulator/1(VdVq_mes)
  Vdc_mes/1 -> VDC Regulator/1(Vdc_mes)
  Vabc_prim/1 -> PLL & Measurements/1(Vabc_prim)
  Iabc_prim/1 -> PLL & Measurements/2(Iabc_prim)
  Unit Delay/1 -> PWM  Generator/1
  PWM  Generator/1 -> Pulses/1
  Uabc_ref Generation  max (m) = 1/1(Uabc_ref) -> Unit Delay/1
  PWM  Generator/2 -> Terminator1/1
  Vdc_ref1/1 -> VDC Regulator/2(Vdc_ref)

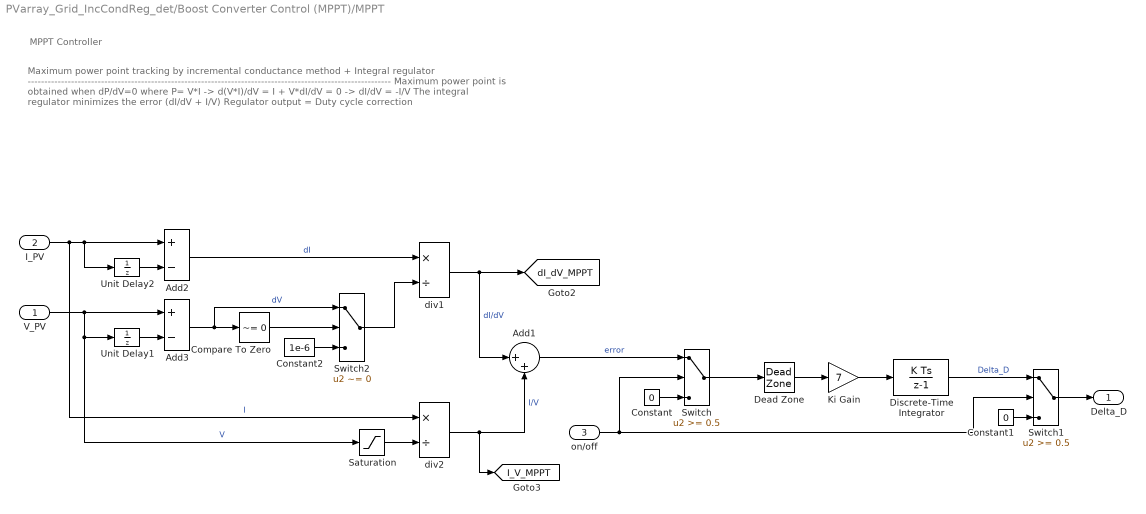
== system PVarray_Grid_IncCondReg_det/Boost Converter Control (MPPT)/MPPT ==
  note: Maximum power point tracking by incremental conductance method + Integral regulator
      | -------------------------------------------------------------------------------------------------------------
      | Maximum power point is obtained when dP/dV=0  where P= V*I
      | -> d(V*I)/dV = I + V*dI/dV = 0
      | -> dI/dV = -I/V
      | The integral regulator minimizes the error (dI/dV + I/V)
      | Regulator output = Duty cycle correction
  note: MPPT Controller
  V_PV : Inport
  I_PV : Inport  Port=2
  on/off : Inport  Port=3
  Add1 : Sum  Inputs=|++
  Add2 : Sum  Inputs=+-
  Add3 : Sum  Inputs=+-
  Compare To Zero : simulink/Logic and Bit Operations/Compare To Zero  relop=~=  OutDataTypeStr=uint8
  Constant : Constant  Value=0
  Constant1 : Constant  Value=0
  Constant2 : Constant  Value=1e-6
  Dead Zone : DeadZone  LowerValue=-0.02  UpperValue=+0.02  SaturateOnIntegerOverflow=on
  Discrete-Time Integrator : DiscreteIntegrator  gainval=1  SampleTime=Ts_Control  LimitOutput=on  UpperSaturationLimit=1  LowerSaturationLimit=-1  ICPrevOutput=DiscIntNeverNeededParam  ICPrevScaledInput=DiscIntNeverNeededParam
  Ki Gain : Gain  Gain=7
  Saturation : Saturate  UpperLimit=inf  LowerLimit=eps
  Switch : Switch  Threshold=0.5
  Switch1 : Switch  Threshold=0.5
  Switch2 : Switch  Criteria=u2 ~= 0
  Unit Delay1 : UnitDelay  SampleTime=Ts_Control  HasFrameUpgradeWarning=on
  Unit Delay2 : UnitDelay  SampleTime=Ts_Control  HasFrameUpgradeWarning=on
  div1 : Product  Inputs=*/  RndMeth=Zero
  div2 : Product  Inputs=*/  RndMeth=Zero
  Delta_D : Outport
  tag scope: I_V_MPPT=global, dI_dV_MPPT=global
  wires:
  V_PV/1 -> Add3/1, Saturation/1, Unit Delay1/1  "V"
  div1/1 -> [dI_dV_MPPT], Add1/1  "dI/dV"
  Constant/1 -> Switch/3
  Switch/1 -> Dead Zone/1
  Unit Delay1/1 -> Add3/2
  Compare To Zero/1 -> Switch2/2
  Switch2/1 -> div1/2
  Constant2/1 -> Switch2/3
  I_PV/1 -> Unit Delay2/1, Add2/1, div2/1  "I"
  Unit Delay2/1 -> Add2/2
  Add3/1 -> Compare To Zero/1, Switch2/1  "dV"
  Add2/1 -> div1/1  "dI"
  Saturation/1 -> div2/2
  div2/1 -> Add1/2, [I_V_MPPT]  "I/V"
  Add1/1 -> Switch/1  "error"
  Dead Zone/1 -> Ki Gain/1
  Constant1/1 -> Switch1/3
  Discrete-Time Integrator/1 -> Switch1/1  "Delta_D"
  Switch1/1 -> Delta_D/1
  on/off/1 -> Switch/2, Switch1/2
  Ki Gain/1 -> Discrete-Time Integrator/1

== system PVarray_Grid_IncCondReg_det/Boost Converter Control (MPPT)/Pulse Generator ==
  D : Inport
  Relational Operator : RelationalOperator  Operator=<=  OutDataTypeStr=boolean  RndMeth=Nearest
  Repeating Sequence : simulink/Sources/Repeating Sequence  rep_seq_t="[0  1/Freq]"  rep_seq_y=[0 1]
  Pulses : Outport
  wires:
  D/1 -> Relational Operator/2
  Relational Operator/1 -> Pulses/1
  Repeating Sequence/1 -> Relational Operator/1

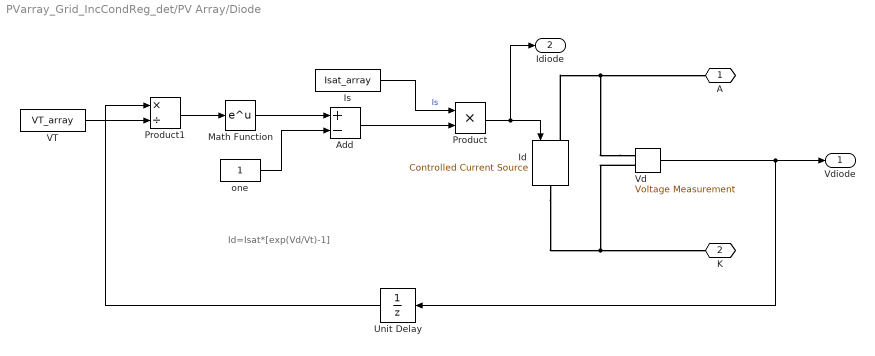
== system PVarray_Grid_IncCondReg_det/PV Array/Diode ==
  note: Id=Isat*[exp(Vd/Vt)-1]
  Add : Sum  Inputs=+-
  Id : powerlib/Electrical Sources/Controlled Current Source  Initialize=on  Source_Type=AC  Amplitude=0  Phase=0  Frequency=0  Measurements=None
  Is : Constant  Value=Isat_array
  Math Function : Math  SignedPower=on  SaturateOnIntegerOverflow=on
  Product : Product  RndMeth=Zero
  Product1 : Product  Inputs=*/  RndMeth=Zero
  Unit Delay : UnitDelay  SampleTime=Ts  HasFrameUpgradeWarning=on
  VT : Constant  Value=VT_array
  Vd : powerlib/Measurements/Voltage Measurement  PhasorSimulation=off  OutputType=Complex  PSBequivalent=0
  one : Constant
  A : PMIOPort  Side=Left
  K : PMIOPort  Port=2  Side=Right
  Vdiode : Outport
  Idiode : Outport  Port=2
  wires:
  Product/1 -> Idiode/1, Id/1
  Vd/1 -> Vdiode/1, Unit Delay/1
  Is/1 -> Product/1  "Is"
  Product1/1 -> Math Function/1
  one/1 -> Add/2
  Add/1 -> Product/2
  VT/1 -> Product1/2
  Unit Delay/1 -> Product1/1
  Math Function/1 -> Add/1
  connections:
  Id/RConn1 -- K/RConn1 -- Vd/LConn2
  Vd/LConn1 -- A/RConn1 -- Id/LConn1

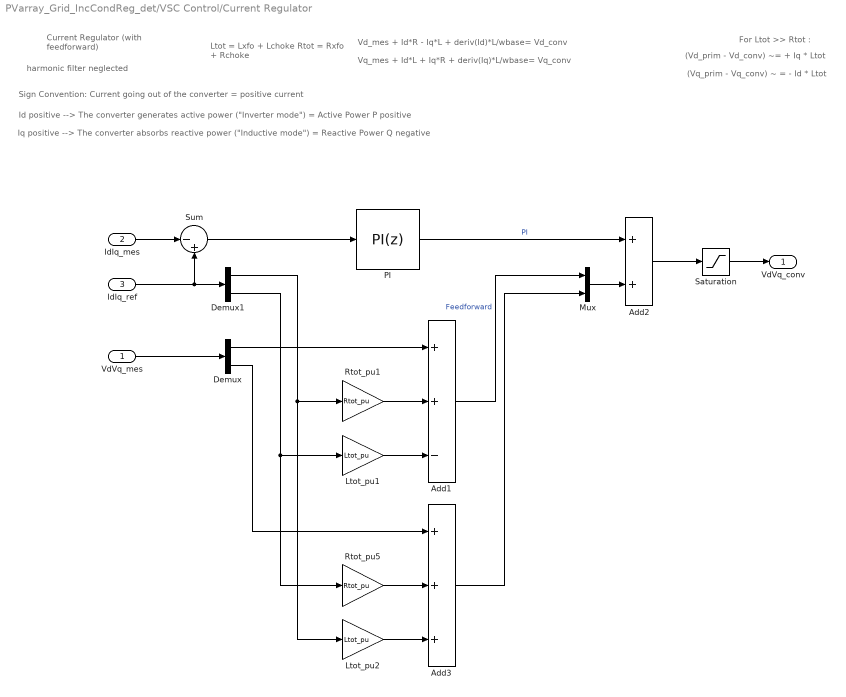
== system PVarray_Grid_IncCondReg_det/VSC Control/Current Regulator ==
  note: harmonic filter neglected
  note: Vd_mes + Id*R - Iq*L + deriv(Id)*L/wbase= Vd_conv
  note: Vq_mes + Id*L + Iq*R + deriv(Iq)*L/wbase= Vq_conv
  note: Current Regulator
      | (with feedforward)
  note: Sign Convention: Current going out of the converter = positive current
  note: Iq positive --> The converter absorbs reactive power ("Inductive mode") = Reactive Power Q negative
  note: Id positive --> The converter generates active power ("Inverter mode") = Active Power P positive
  note: Ltot = Lxfo + Lchoke
      | Rtot = Rxfo + Rchoke
  note: (Vd_prim - Vd_conv) ~= + Iq * Ltot
  note: (Vq_prim - Vq_conv) ~ = - Id * Ltot
  note: For Ltot >> Rtot :
  VdVq_mes : Inport  PortDimensions=2
  IdIq_mes : Inport  Port=2  PortDimensions=2
  IdIq_ref : Inport  Port=3  PortDimensions=2
  Add1 : Sum  Inputs=++-
  Add2 : Sum
  Add3 : Sum  Inputs=+++
  Demux : Demux  Outputs=2
  Demux1 : Demux  Outputs=2
  Ltot_pu1 : Gain  Gain=Ltot_pu  SaturateOnIntegerOverflow=on  OutDataTypeStr=Inherit: Same as input  ParamDataTypeStr=Inherit: Same as input
  Ltot_pu2 : Gain  Gain=Ltot_pu  SaturateOnIntegerOverflow=on  OutDataTypeStr=Inherit: Same as input  ParamDataTypeStr=Inherit: Same as input
  Mux : Mux  Inputs=2
  PI : simulink/Continuous/PID Controller  Controller=PI  Form=Parallel  TimeDomain=Discrete-time  UseExternalTs=off  SampleTime=Ts  IntegratorMethod=Forward Euler  FilterMethod=Forward Euler  ControllerParametersSource=internal  P=Kp_Ireg  I=Ki_Ireg  D=0  UseFilter=on  N=100  TunerSelectOption=Transfer Function Based (PID Tuner App)  InitialConditionSource=internal  InitialConditionForIntegrator=0  InitialConditionForFilter=0  DifferentiatorICPrevScaledInput=0  ExternalReset=none  TrackingMode=off  Kt=1  LimitOutput=on  UpperSaturationLimit=2  LowerSaturationLimit=-2  LinearizeAsGain=off  AntiWindupMode=none  Kb=1  POutMin=[]  POutMax=[]  IOutMin=[]  IOutMax=[]  DOutMin=[]  DOutMax=[]  NOutMin=[]  NOutMax=[]  SumOutMin=[]  SumOutMax=[]  SaturationOutMin=[]  SaturationOutMax=[]  PParamMin=[]  PParamMax=[]  IParamMin=[]  IParamMax=[]  DParamMin=[]  DParamMax=[]  NParamMin=[]  NParamMax=[]  KbParamMin=[]  KbParamMax=[]  KtParamMin=[]  KtParamMax=[]  KbOutMin=[]  KbOutMax=[]  KtOutMin=[]  KtOutMax=[]  IntegratorOutMin=[]  IntegratorOutMax=[]  FilterOutMin=[]  FilterOutMax=[]  SumI1OutMin=[]  SumI1OutMax=[]  SumI2OutMin=[]  SumI2OutMax=[]  SumI3OutMin=[]  SumI3OutMax=[]  SumI4OutMin=[]  SumI4OutMax=[]  SumDOutMin=[]  SumDOutMax=[]  DifferentiatorOutMin=[]  DifferentiatorOutMax=[]  FilterDiffOutCoefMin=[]  FilterDiffOutCoefMax=[]  ReciprocalOutMin=[]  ReciprocalOutMax=[]  SumDenOutMin=[]  SumDenOutMax=[]  SumNumOutMin=[]  SumNumOutMax=[]  DivideOutMin=[]  DivideOutMax=[]  UdiffTsProdOutMin=[]  UdiffTsProdOutMax=[]  NTsProdOutMin=[]  NTsProdOutMax=[]  UintegralTsProdOutMin=[]  UintegralTsProdOutMax=[]  UngainTsProdOutMin=[]  UngainTsProdOutMax=[]  IntegratorContinuousStateAttributes=''  IntegratorStateMustResolveToSignalObject=off  IntegratorRTWStateStorageClass=Auto  FilterContinuousStateAttributes=''  FilterStateMustResolveToSignalObject=off  FilterRTWStateStorageClass=Auto  ParallelPVariant=InternalParameters  IdealPVariant=Disabled  IVariant=InternalParameters  DVariant=Disabled  IntegratorVariant=Discrete  SatVariant=Enabled  AWVariant=Passthrough  PCopyVariant=Disabled  TRVariant=Disabled  FdbkBlocksVariant=Forward  IdealPFdbkVariant=Disabled  SatFdbkVariant=Disabled  DerivativeFilterVariant=Disabled  NVariant=Disabled  NCopyVariant=Disabled_SignalSpec  FilterICVariant=Disabled  IntegratorICVariant=InternalICs  ExternalResetVariant=Disabled  TRSumVariant=Passthrough  SumFdbkVariant=Disabled  SumVariant=Sum_PI  TsampFilterVariant=InternalTs  TsampNgainVariant=Passthrough  TsampIntegralVariant=Passthrough
  Rtot_pu1 : Gain  Gain=Rtot_pu  SaturateOnIntegerOverflow=on  OutDataTypeStr=Inherit: Same as input  ParamDataTypeStr=Inherit: Same as input
  Rtot_pu5 : Gain  Gain=Rtot_pu  SaturateOnIntegerOverflow=on  OutDataTypeStr=Inherit: Same as input  ParamDataTypeStr=Inherit: Same as input
  Saturation : Saturate  UpperLimit=2  LowerLimit=-2
  Sum : Sum  Inputs=|-+
  VdVq_conv : Outport
  wires:
  Mux/1 -> Add2/2
  PI/1 -> Add2/1  "PI"
  Sum/1 -> PI/1
  IdIq_ref/1 -> Sum/2, Demux1/1
  IdIq_mes/1 -> Sum/1
  Add2/1 -> Saturation/1
  Saturation/1 -> VdVq_conv/1
  VdVq_mes/1 -> Demux/1
  Demux/1 -> Add1/1
  Rtot_pu1/1 -> Add1/2
  Demux1/1 -> Rtot_pu1/1, Ltot_pu2/1
  Ltot_pu1/1 -> Add1/3
  Demux1/2 -> Ltot_pu1/1, Rtot_pu5/1
  Rtot_pu5/1 -> Add3/2
  Ltot_pu2/1 -> Add3/3
  Add1/1 -> Mux/1  "Feedforward"
  Demux/2 -> Add3/1
  Add3/1 -> Mux/2

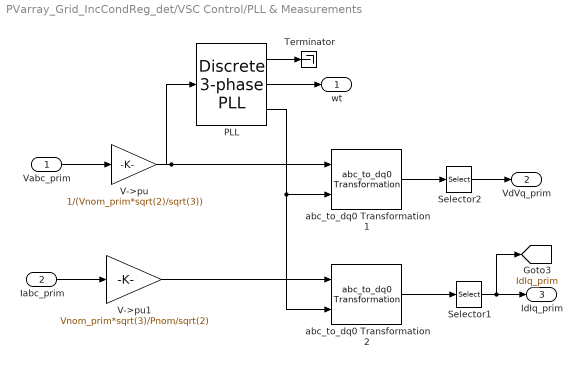
== system PVarray_Grid_IncCondReg_det/VSC Control/PLL & Measurements ==
  Vabc_prim : Inport
  Iabc_prim : Inport  Port=2
  PLL : powerlib_extras/Discrete  Control Blocks/Discrete 3-phase PLL  Fmin=45  Par_Init="[-0.57  Fnom]"  ParK=[60 1400]  Ts=Ts  AGC=off
      settings: SourceProductBaseCode=PS
  Selector1 : Selector  InputPortWidth=3  IndexOptions=Index vector (dialog)  Indices=[1 2]  OutputSizes=1
  Selector2 : Selector  InputPortWidth=3  IndexOptions=Index vector (dialog)  Indices=[1 2]  OutputSizes=1
  Terminator : Terminator
  V->pu : Gain  Gain=1/(Vnom_prim*sqrt(2)/sqrt(3))  SaturateOnIntegerOverflow=on  OutDataTypeStr=Inherit: Same as input  ParamDataTypeStr=Inherit: Same as input
  V->pu1 : Gain  Gain=Vnom_prim*sqrt(3)/Pnom/sqrt(2)  SaturateOnIntegerOverflow=on  OutDataTypeStr=Inherit: Same as input  ParamDataTypeStr=Inherit: Same as input
  abc_to_dq0 Transformation1 : powerlib_extras/Measurements/abc_to_dq0 Transformation
      settings: SourceProductBaseCode=PS
  abc_to_dq0 Transformation2 : powerlib_extras/Measurements/abc_to_dq0 Transformation
      settings: SourceProductBaseCode=PS
  wt : Outport
  VdVq_prim : Outport  Port=2
  IdIq_prim : Outport  Port=3
  tag scope: IdIq_prim=global
  wires:
  V->pu1/1 -> abc_to_dq0 Transformation2/1
  V->pu/1 -> PLL/1, abc_to_dq0 Transformation1/1
  abc_to_dq0 Transformation2/1 -> Selector1/1
  PLL/2 -> wt/1
  Vabc_prim/1 -> V->pu/1
  Iabc_prim/1 -> V->pu1/1
  abc_to_dq0 Transformation1/1 -> Selector2/1
  Selector2/1 -> VdVq_prim/1
  Selector1/1 -> [IdIq_prim], IdIq_prim/1
  PLL/3 -> abc_to_dq0 Transformation2/2, abc_to_dq0 Transformation1/2
  PLL/1 -> Terminator/1

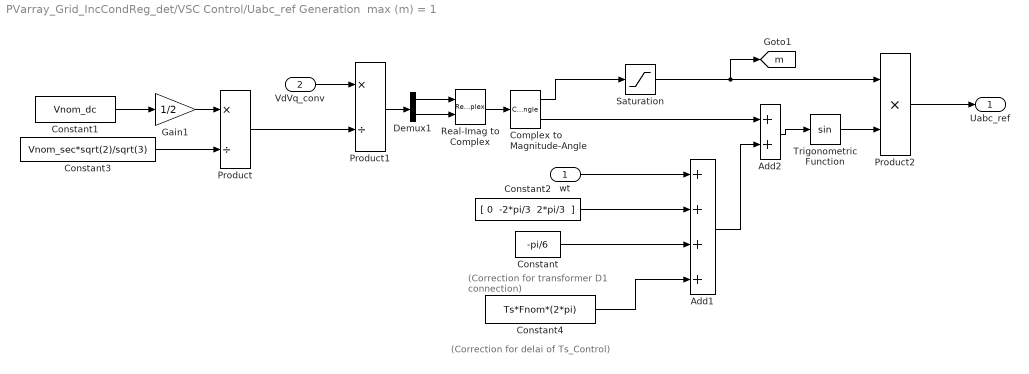
== system PVarray_Grid_IncCondReg_det/VSC Control/Uabc_ref Generation  max (m) = 1 ==
  note: (Correction for transformer
      |  D1 connection)
  note: (Correction for delai of Ts_Control)
  wt : Inport
  VdVq_conv : Inport  Port=2
  Add1 : Sum  Inputs=++++
  Add2 : Sum
  Complex to Magnitude-Angle : ComplexToMagnitudeAngle
  Constant : Constant  Value=-pi/6
  Constant1 : Constant  Value=Vnom_dc
  Constant2 : Constant  Value="[ 0  -2*pi/3  2*pi/3  ]"
  Constant3 : Constant  Value=Vnom_sec*sqrt(2)/sqrt(3)
  Constant4 : Constant  Value=Ts*Fnom*(2*pi)
  Demux1 : Demux  Outputs=2
  Gain1 : Gain  Gain=1/2
  Product : Product  Inputs=*/  RndMeth=Zero
  Product1 : Product  Inputs=*/  RndMeth=Zero
  Product2 : Product  Inputs=**  RndMeth=Zero
  Real-Imag to Complex : RealImagToComplex
  Saturation : Saturate  UpperLimit=1  LowerLimit=0
  Trigonometric Function : Trigonometry
  Uabc_ref : Outport
  tag scope: m=global
  wires:
  Complex to Magnitude-Angle/1 -> Saturation/1
  Constant1/1 -> Gain1/1
  VdVq_conv/1 -> Product1/1
  Product1/1 -> Demux1/1
  Gain1/1 -> Product/1
  Real-Imag to Complex/1 -> Complex to Magnitude-Angle/1
  Demux1/1 -> Real-Imag to Complex/1
  Demux1/2 -> Real-Imag to Complex/2
  Constant2/1 -> Add1/2
  Constant/1 -> Add1/3
  Constant3/1 -> Product/2
  Product/1 -> Product1/2
  Complex to Magnitude-Angle/2 -> Add2/1
  Add1/1 -> Add2/2
  Add2/1 -> Trigonometric Function/1
  Saturation/1 -> [m], Product2/1
  Trigonometric Function/1 -> Product2/2
  Product2/1 -> Uabc_ref/1
  wt/1 -> Add1/1
  Constant4/1 -> Add1/4

== system PVarray_Grid_IncCondReg_det/VSC Control/VDC Regulator ==
  Vdc_mes : Inport  PortDimensions=1
  Vdc_ref : Inport  Port=2  PortDimensions=1
  PI : simulink/Continuous/PID Controller  Controller=PI  Form=Parallel  TimeDomain=Discrete-time  UseExternalTs=off  SampleTime=Ts  IntegratorMethod=Trapezoidal  FilterMethod=Forward Euler  ControllerParametersSource=internal  P=Kp_VDCreg  I=Ki_VDCreg  D=0  UseFilter=on  N=100  TunerSelectOption=Transfer Function Based (PID Tuner App)  InitialConditionSource=internal  InitialConditionForIntegrator=0  InitialConditionForFilter=0  DifferentiatorICPrevScaledInput=0  ExternalReset=none  TrackingMode=off  Kt=1  LimitOutput=on  UpperSaturationLimit=1.5  LowerSaturationLimit=-1.5  LinearizeAsGain=off  AntiWindupMode=none  Kb=1  POutMin=[]  POutMax=[]  IOutMin=[]  IOutMax=[]  DOutMin=[]  DOutMax=[]  NOutMin=[]  NOutMax=[]  SumOutMin=[]  SumOutMax=[]  SaturationOutMin=[]  SaturationOutMax=[]  PParamMin=[]  PParamMax=[]  IParamMin=[]  IParamMax=[]  DParamMin=[]  DParamMax=[]  NParamMin=[]  NParamMax=[]  KbParamMin=[]  KbParamMax=[]  KtParamMin=[]  KtParamMax=[]  KbOutMin=[]  KbOutMax=[]  KtOutMin=[]  KtOutMax=[]  IntegratorOutMin=[]  IntegratorOutMax=[]  FilterOutMin=[]  FilterOutMax=[]  SumI1OutMin=[]  SumI1OutMax=[]  SumI2OutMin=[]  SumI2OutMax=[]  SumI3OutMin=[]  SumI3OutMax=[]  SumI4OutMin=[]  SumI4OutMax=[]  SumDOutMin=[]  SumDOutMax=[]  DifferentiatorOutMin=[]  DifferentiatorOutMax=[]  FilterDiffOutCoefMin=[]  FilterDiffOutCoefMax=[]  ReciprocalOutMin=[]  ReciprocalOutMax=[]  SumDenOutMin=[]  SumDenOutMax=[]  SumNumOutMin=[]  SumNumOutMax=[]  DivideOutMin=[]  DivideOutMax=[]  UdiffTsProdOutMin=[]  UdiffTsProdOutMax=[]  NTsProdOutMin=[]  NTsProdOutMax=[]  UintegralTsProdOutMin=[]  UintegralTsProdOutMax=[]  UngainTsProdOutMin=[]  UngainTsProdOutMax=[]  IntegratorContinuousStateAttributes=''  IntegratorStateMustResolveToSignalObject=off  IntegratorRTWStateStorageClass=Auto  FilterContinuousStateAttributes=''  FilterStateMustResolveToSignalObject=off  FilterRTWStateStorageClass=Auto  ParallelPVariant=InternalParameters  IdealPVariant=Disabled  IVariant=InternalParameters  DVariant=Disabled  IntegratorVariant=Discrete  SatVariant=Enabled  AWVariant=Passthrough  PCopyVariant=Disabled  TRVariant=Disabled  FdbkBlocksVariant=Forward  IdealPFdbkVariant=Disabled  SatFdbkVariant=Disabled  DerivativeFilterVariant=Disabled  NVariant=Disabled  NCopyVariant=Disabled_SignalSpec  FilterICVariant=Disabled  IntegratorICVariant=InternalICs  ExternalResetVariant=Disabled  TRSumVariant=Passthrough  SumFdbkVariant=Disabled  SumVariant=Sum_PI  TsampFilterVariant=InternalTs  TsampNgainVariant=Passthrough  TsampIntegralVariant=Passthrough
  Rtot_pu3 : Gain  Gain=1/Vnom_dc  SaturateOnIntegerOverflow=on  OutDataTypeStr=Inherit: Same as input  ParamDataTypeStr=Inherit: Same as input
  Sum : Sum  Inputs=|+-
  Id_ref : Outport  SampleTime=Ts  InitialOutput=0
  tag scope: Id_ref=global, Vdc_ref=global
  wires:
  Sum/1 -> Rtot_pu3/1
  Vdc_mes/1 -> Sum/1
  Vdc_ref/1 -> Sum/2, [Vdc_ref]
  Rtot_pu3/1 -> PI/1
  PI/1 -> [Id_ref], Id_ref/1
